simulink model "CLSfixedExample1"  (R2025b)
settings: Solver=FixedStepAuto  StartTime=0.0  StopTime=10  FixedStep=0.0005  RelTol=1e-3
undefined symbols (not defined in the file): AVI, BCL, cfg_length, f1, f2, LRI, pNode_length, pPath_length, PVARP, SD, sig1, sig2, stepsize, URI, VR, VRP, VT
libraries: Libs x8, Libs_unified x3
settings Model: SimulationMode=accelerator  Creator=ball907  LastModifiedBy=rfen801
settings SolverCC: AutoInsertRateTranBlk=on
settings OptimizationCC: DefaultParameterBehavior=Inlined
settings ModelReferenceCC: EnableRefExpFcnMdlSchedulingChecks=on
settings RTWCC: Toolchain=Simulink Real-Time Toolchain  BuildConfiguration=Faster Runs  CodeExecutionProfiling=on

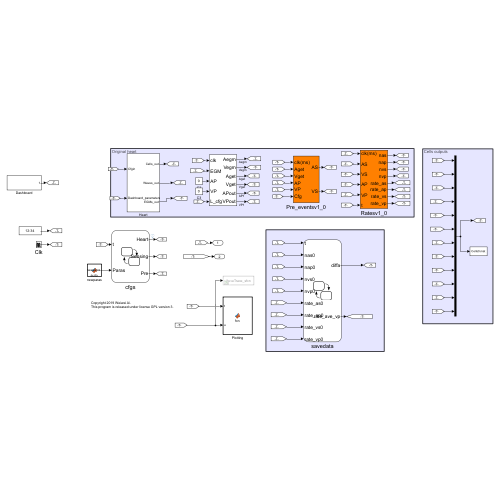
[thumbnail: Simulink's stored preview of the top-level diagram]
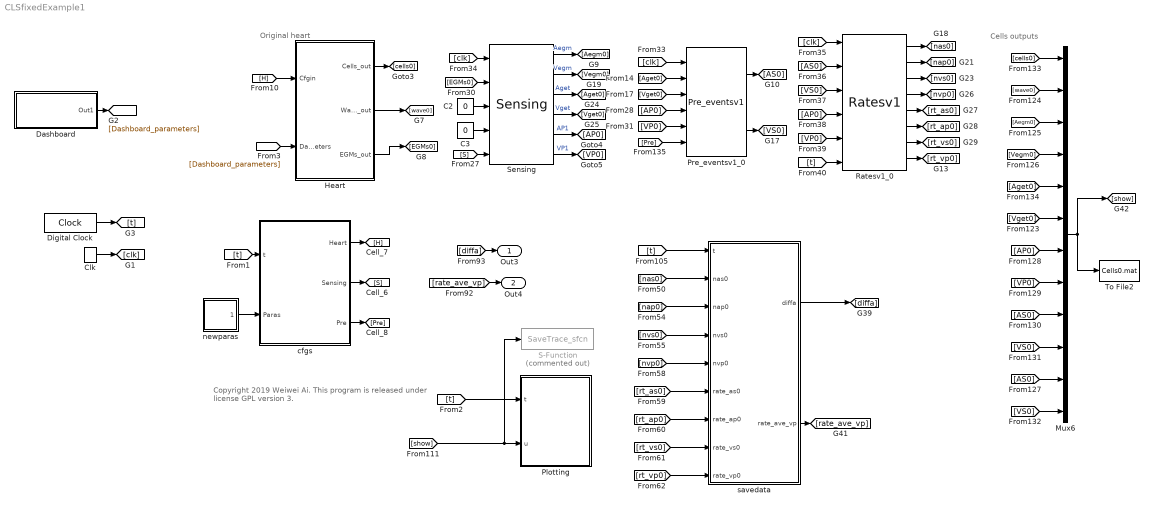
== system CLSfixedExample1 ==
  note: Cells outputs
  note: Copyright 2019 Weiwei Ai.
      | This program is released under license GPL version 3.
  note: Original heart
  C2 : Constant  Value=0
  C3 : Constant  Value=0
  Clk : DiscretePulseGenerator  PulseType=Time based  Period=1  PulseWidth=50
  Dashboard : Subsystem
  Digital Clock : DigitalClock  SampleTime=stepsize
  Heart : Subsystem
  Mux6 : Mux  Inputs=12
  Plotting : MATLAB Function  TreatAsAtomicUnit=on  SystemSampleTime=stepsize*5
  Pre_eventsv1_0 : Libs_unified/Pre_eventsv1  SystemSampleTime=-1  VariantActivationTime=update diagram  EmptyChoice=off  PassThrough=off  PassThroughVariantControl=(default)  EmptyChoiceVariantControl=(default)  AllowFlexibleInterface=on  Latency=0  AutoFrameSizeCalculation=off
  Ratesv1_0 : Libs_unified/Ratesv1  SystemSampleTime=-1  VariantActivationTime=update diagram  EmptyChoice=off  PassThrough=off  PassThroughVariantControl=(default)  EmptyChoiceVariantControl=(default)  AllowFlexibleInterface=on  Latency=0  AutoFrameSizeCalculation=off
  S-Function : S-Function  Commented=on  FunctionName=SaveTrace_sfcn  Parameters=1  SFunctionDeploymentMode=off  EnableBusSupport=off
  Sensing : Libs_unified/Sensing  SystemSampleTime=-1  VariantActivationTime=update diagram  EmptyChoice=off  PassThrough=off  PassThroughVariantControl=(default)  EmptyChoiceVariantControl=(default)  AllowFlexibleInterface=on  Latency=0  AutoFrameSizeCalculation=off
  To File2 : ToFile  Filename=Cells0.mat  MatrixName=cells
      settings: Decimation=2
  cfgs : Stateflow chart  TreatAsAtomicUnit=on
  newparas : MATLAB Function  TreatAsAtomicUnit=on
  savedata : Stateflow chart  TreatAsAtomicUnit=on
  Out3 : Outport
  Out4 : Outport  Port=2
  wires:
  Sensing/6 -> [VP0]  "VP1"
  [VS0] -> Mux6/10
  [VS0] -> Ratesv1_0/3
  Pre_eventsv1_0/1 -> [AS0]
  [nap0] -> savedata/3(nap0)
  [VP0] -> Pre_eventsv1_0/5
  [AS0] -> Mux6/11
  Sensing/3 -> [Aget0]  "Aget"
  [rt_ap0] -> savedata/7(rate_ap0)
  C3/1 -> Sensing/4
  [AS0] -> Mux6/9
  Sensing/1 -> [Aegm0]  "Aegm"
  Ratesv1_0/4 -> [nvp0]
  [t] -> savedata/1(t)
  savedata/1(diffa) -> [diffa]
  Heart/3(EGMs_out) -> [EGMs0]
  [cells0] -> Mux6/1
  Pre_eventsv1_0/2 -> [VS0]
  Sensing/4 -> [Vget0]  "Vget"
  Ratesv1_0/5 -> [rt_as0]
  Ratesv1_0/3 -> [nvs0]
  [rt_vp0] -> savedata/9(rate_vp0)
  [rt_vs0] -> savedata/8(rate_vs0)
  [Aget0] -> Pre_eventsv1_0/2
  Sensing/5 -> [AP0]  "AP1"
  Ratesv1_0/1 -> [nas0]
  [diffa] -> Out3/1
  Heart/1(Cells_out) -> [cells0]
  Ratesv1_0/2 -> [nap0]
  [VP0] -> Mux6/8
  Mux6/1 -> [show], To File2/1
  [AS0] -> Ratesv1_0/2
  [AP0] -> Mux6/7
  [t] -> Ratesv1_0/6
  [Aegm0] -> Mux6/3
  [nvs0] -> savedata/4(nvs0)
  [Vget0] -> Mux6/6
  [rt_as0] -> savedata/6(rate_as0)
  [VS0] -> Mux6/12
  [AP0] -> Ratesv1_0/4
  Heart/2(Waves_out) -> [wave0]
  [clk] -> Ratesv1_0/1
  [clk] -> Pre_eventsv1_0/1
  [Pre] -> Pre_eventsv1_0/6
  [Vget0] -> Pre_eventsv1_0/3
  [wave0] -> Mux6/2
  [VP0] -> Ratesv1_0/5
  [AP0] -> Pre_eventsv1_0/4
  savedata/2(rate_ave_vp) -> [rate_ave_vp]
  C2/1 -> Sensing/3
  [S] -> Sensing/5
  [rate_ave_vp] -> Out4/1
  Ratesv1_0/7 -> [rt_vs0]
  [Vegm0] -> Mux6/4
  [clk] -> Sensing/1
  Ratesv1_0/8 -> [rt_vp0]
  [Aget0] -> Mux6/5
  [nas0] -> savedata/2(nas0)
  [EGMs0] -> Sensing/2
  Sensing/2 -> [Vegm0]  "Vegm"
  Ratesv1_0/6 -> [rt_ap0]
  [nvp0] -> savedata/5(nvp0)
  cfgs/2(Sensing) -> [S]
  cfgs/3(Pre) -> [Pre]
  newparas/1(newparas) -> cfgs/2(Paras)
  cfgs/1(Heart) -> [H]
  [t] -> cfgs/1(t)
  Digital Clock/1 -> [t]
  Clk/1 -> [clk]
  [show] -> S-Function/1, Plotting/2(u)
  [t] -> Plotting/1(t)
  [H] -> Heart/1(Cfgin)
  [Dashboard_parameters] -> Heart/2(Dashboard_parameters)
  Dashboard/1(Out1) -> [Dashboard_parameters]

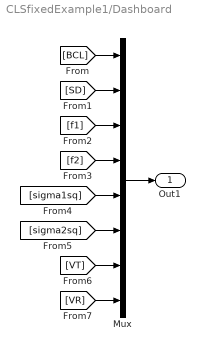
== system CLSfixedExample1/Dashboard ==
  Mux : Mux  Inputs=8
  Out1 : Outport
  wires:
  Mux/1 -> Out1/1
  [BCL] -> Mux/1
  [SD] -> Mux/2
  [f1] -> Mux/3
  [f2] -> Mux/4
  [sigma1sq] -> Mux/5
  [sigma2sq] -> Mux/6
  [VT] -> Mux/7
  [VR] -> Mux/8

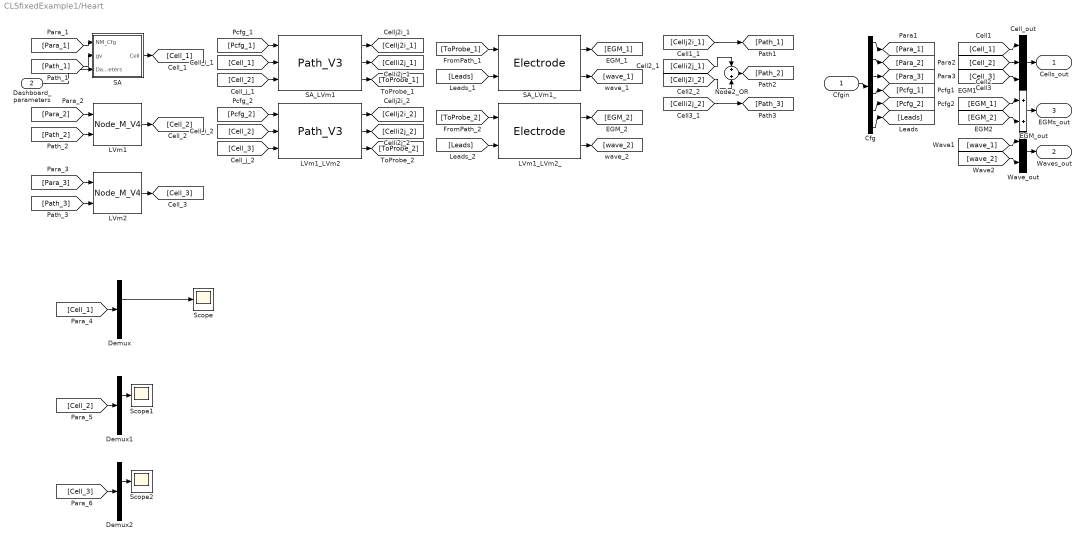
== system CLSfixedExample1/Heart ==
  Cfgin : Inport
  Dashboard_parameters : Inport  Port=2
  Cell_out : Mux  Inputs=3
  Cfg : Demux  Outputs=[50,25,25,11,11,28]
  Demux : Demux  Outputs=5
  Demux1 : Demux  Outputs=5
  Demux2 : Demux  Outputs=5
  EGM_out : Sum  Inputs=2
  LVm1 : Libs/Node_M_V4  SystemSampleTime=-1  VariantActivationTime=update diagram  EmptyChoice=off  PassThrough=off  PassThroughVariantControl=(default)  EmptyChoiceVariantControl=(default)  AllowFlexibleInterface=on  Latency=0  AutoFrameSizeCalculation=off
  LVm1_LVm2 : Libs/Path_V3  SystemSampleTime=-1  VariantActivationTime=update diagram  EmptyChoice=off  PassThrough=off  PassThroughVariantControl=(default)  EmptyChoiceVariantControl=(default)  AllowFlexibleInterface=on  Latency=0  AutoFrameSizeCalculation=off
  LVm1_LVm2_ : Libs/Electrode  SystemSampleTime=-1  VariantActivationTime=update diagram  EmptyChoice=off  PassThrough=off  PassThroughVariantControl=(default)  EmptyChoiceVariantControl=(default)  AllowFlexibleInterface=on  Latency=0  AutoFrameSizeCalculation=off
  LVm2 : Libs/Node_M_V4  SystemSampleTime=-1  VariantActivationTime=update diagram  EmptyChoice=off  PassThrough=off  PassThroughVariantControl=(default)  EmptyChoiceVariantControl=(default)  AllowFlexibleInterface=on  Latency=0  AutoFrameSizeCalculation=off
  Node2_OR : Sum  Inputs=2
  SA : Subsystem  AncestorBlock=Libs/Node_NM_V4
  SA_LVm1 : Libs/Path_V3  SystemSampleTime=-1  VariantActivationTime=update diagram  EmptyChoice=off  PassThrough=off  PassThroughVariantControl=(default)  EmptyChoiceVariantControl=(default)  AllowFlexibleInterface=on  Latency=0  AutoFrameSizeCalculation=off
  SA_LVm1_ : Libs/Electrode  SystemSampleTime=-1  VariantActivationTime=update diagram  EmptyChoice=off  PassThrough=off  PassThroughVariantControl=(default)  EmptyChoiceVariantControl=(default)  AllowFlexibleInterface=on  Latency=0  AutoFrameSizeCalculation=off
  Scope : Scope
      settings: ActiveDisplayYMinimum=-15.358773094825372  ActiveDisplayYMaximum=138.22895785342837
  Scope1 : Scope
      settings: ActiveDisplayYMinimum=-15.358773094825372  ActiveDisplayYMaximum=138.22895785342837
  Scope2 : Scope
      settings: ActiveDisplayYMinimum=-15.358773094825372  ActiveDisplayYMaximum=138.22895785342837  DataLoggingVariableName=ScopeData2
  Wave_out : Mux  Inputs=2
  Cells_out : Outport
  Waves_out : Outport  Port=2
  EGMs_out : Outport  Port=3
  wires:
  [wave_2] -> Wave_out/2
  [wave_1] -> Wave_out/1
  [EGM_2] -> EGM_out/2
  [EGM_1] -> EGM_out/1
  [Cell_3] -> Cell_out/3
  [Cell_2] -> Cell_out/2
  [Cell_1] -> Cell_out/1
  Wave_out/1 -> Waves_out/1
  EGM_out/1 -> EGMs_out/1
  Cell_out/1 -> Cells_out/1
  Cfg/6 -> [Leads]
  Cfg/5 -> [Pcfg_2]
  Cfg/4 -> [Pcfg_1]
  Cfg/3 -> [Para_3]
  Cfg/2 -> [Para_2]
  Cfg/1 -> [Para_1]
  Cfgin/1 -> Cfg/1
  [Celli2j_2] -> [Path_3]
  Node2_OR/1 -> [Path_2]
  [Cellj2i_2] -> Node2_OR/2
  [Celli2j_1] -> Node2_OR/1
  [Cellj2i_1] -> [Path_1]
  [Leads] -> LVm1_LVm2_/2
  [ToProbe_2] -> LVm1_LVm2_/1
  LVm1_LVm2_/2 -> [wave_2]
  LVm1_LVm2_/1 -> [EGM_2]
  [Leads] -> SA_LVm1_/2
  [ToProbe_1] -> SA_LVm1_/1
  SA_LVm1_/2 -> [wave_1]
  SA_LVm1_/1 -> [EGM_1]
  [Cell_3] -> LVm1_LVm2/3
  [Cell_2] -> LVm1_LVm2/2
  [Pcfg_2] -> LVm1_LVm2/1
  LVm1_LVm2/3 -> [ToProbe_2]
  LVm1_LVm2/2 -> [Celli2j_2]
  LVm1_LVm2/1 -> [Cellj2i_2]
  [Cell_2] -> SA_LVm1/3
  [Cell_1] -> SA_LVm1/2
  [Pcfg_1] -> SA_LVm1/1
  SA_LVm1/3 -> [ToProbe_1]
  SA_LVm1/2 -> [Celli2j_1]
  SA_LVm1/1 -> [Cellj2i_1]
  [Path_3] -> LVm2/2
  [Para_3] -> LVm2/1
  LVm2/1 -> [Cell_3]
  [Path_2] -> LVm1/2
  [Para_2] -> LVm1/1
  LVm1/1 -> [Cell_2]
  [Path_1] -> SA/2(gv)
  [Para_1] -> SA/1(NM_Cfg)
  SA/1(Cell) -> [Cell_1]
  [Cell_1] -> Demux/1
  Demux/2 -> Scope/1
  [Cell_2] -> Demux1/1
  Demux1/2 -> Scope1/1
  [Cell_3] -> Demux2/1
  Demux2/2 -> Scope2/1
  Dashboard_parameters/1 -> SA/3(Dashboard_parameters)

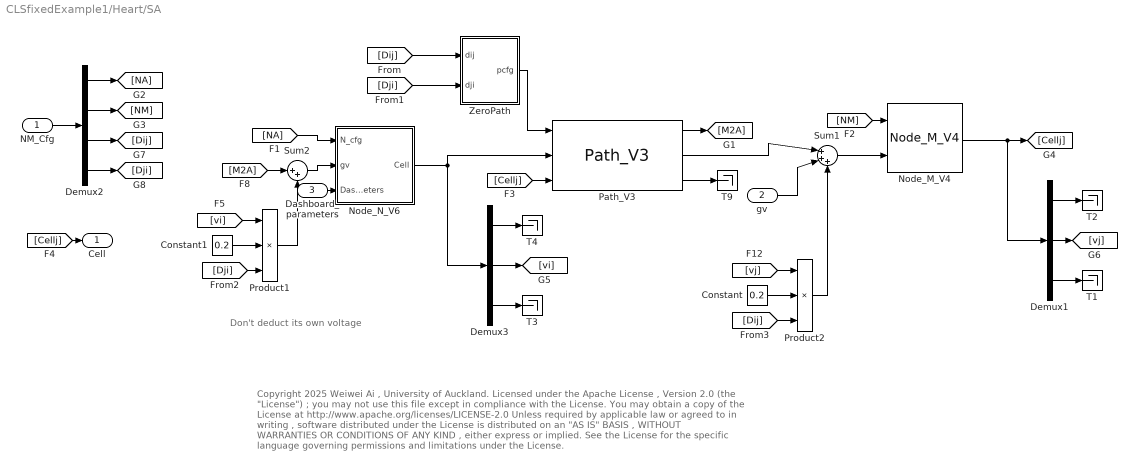
== system CLSfixedExample1/Heart/SA ==
  note: Copyright 2025 Weiwei Ai , University of Auckland.
      | Licensed under the Apache License , Version 2.0 (the "License") ;
      | you may not use this file except in compliance with the License.
      | You may obtain a copy of the License at
      | http://www.apache.org/licenses/LICENSE-2.0
      | Unless required by applicable law or agreed to in writing , software
      | distributed under the License is distributed on an "AS IS" BASIS ,
      | WITHOUT WARRANTIES OR CONDITIONS OF ANY KIND , either express or implied.
      | See the License for the specific language governing permissions and
      | limitations under the License.
  note: Don't deduct its own voltage
  NM_Cfg : Inport
  gv : Inport  Port=2
  Dashboard_parameters : Inport  Port=3
  Constant : Constant  Value=0.2
  Constant1 : Constant  Value=0.2
  Demux1 : Demux  Outputs=[1,1,3]
  Demux2 : Demux  Outputs=[23,25,1,1]
  Demux3 : Demux  Outputs=[1,1,3]
  Node_M_V4 : Libs/Node_M_V4  SystemSampleTime=-1  VariantActivationTime=update diagram  EmptyChoice=off  PassThrough=off  PassThroughVariantControl=(default)  EmptyChoiceVariantControl=(default)  AllowFlexibleInterface=on  Latency=0  AutoFrameSizeCalculation=off
  Node_N_V6 : Subsystem  AncestorBlock=Libs/Node_N_V6
  Path_V3 : Libs/Path_V3  SystemSampleTime=-1  VariantActivationTime=update diagram  EmptyChoice=off  PassThrough=off  PassThroughVariantControl=(default)  EmptyChoiceVariantControl=(default)  AllowFlexibleInterface=on  Latency=0  AutoFrameSizeCalculation=off
  Product1 : Product  Inputs=***
  Product2 : Product  Inputs=***
  Sum1 : Sum  Inputs=|+++
  Sum2 : Sum  Inputs=|++
  T{1..4,9} (5 alike) : Terminator
  ZeroPath : MATLAB Function  TreatAsAtomicUnit=on
  Cell : Outport
  wires:
  [Dij] -> Product2/3
  [Dji] -> Product1/3
  [Dji] -> ZeroPath/2(dji)
  [Dij] -> ZeroPath/1(dij)
  Demux2/4 -> [Dji]
  Demux2/3 -> [Dij]
  Product1/1 -> Sum2/2
  [vi] -> Product1/1
  Constant1/1 -> Product1/2
  Sum2/1 -> Node_N_V6/2(gv)
  [M2A] -> Sum2/1
  gv/1 -> Sum1/2
  Product2/1 -> Sum1/3
  [vj] -> Product2/1
  Constant/1 -> Product2/2
  Demux1/2 -> [vj]
  Demux3/2 -> [vi]
  Demux3/1 -> T4/1
  Demux3/3 -> T3/1
  Node_N_V6/1(Cell) -> Demux3/1, Path_V3/2
  Demux1/1 -> T2/1
  Demux1/3 -> T1/1
  Sum1/1 -> Node_M_V4/2
  Path_V3/2 -> Sum1/1
  ZeroPath/1(pcfg) -> Path_V3/1
  [Cellj] -> Cell/1
  [Cellj] -> Path_V3/3
  Node_M_V4/1 -> [Cellj], Demux1/1
  Path_V3/1 -> [M2A]
  [NM] -> Node_M_V4/1
  [NA] -> Node_N_V6/1(N_cfg)
  Demux2/2 -> [NM]
  Demux2/1 -> [NA]
  Path_V3/3 -> T9/1
  NM_Cfg/1 -> Demux2/1
  Dashboard_parameters/1 -> Node_N_V6/3(Dashboard_parameters)

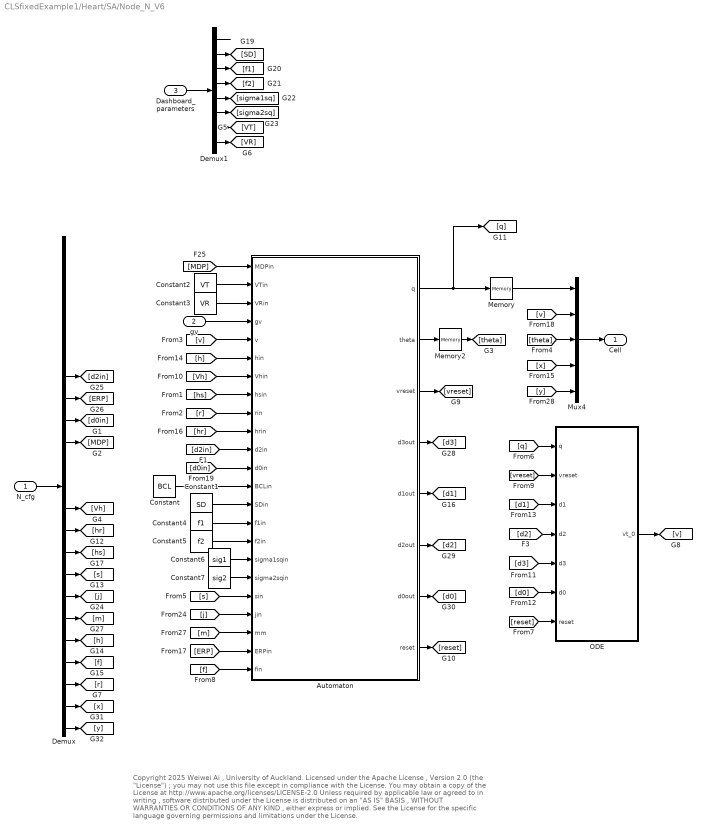
== system CLSfixedExample1/Heart/SA/Node_N_V6 ==
  note: Copyright 2025 Weiwei Ai , University of Auckland.
      | Licensed under the Apache License , Version 2.0 (the "License") ;
      | you may not use this file except in compliance with the License.
      | You may obtain a copy of the License at
      | http://www.apache.org/licenses/LICENSE-2.0
      | Unless required by applicable law or agreed to in writing , software
      | distributed under the License is distributed on an "AS IS" BASIS ,
      | WITHOUT WARRANTIES OR CONDITIONS OF ANY KIND , either express or implied.
      | See the License for the specific language governing permissions and
      | limitations under the License.
  N_cfg : Inport
  gv : Inport  Port=2
  Dashboard_parameters : Inport  Port=3
  Automaton : Stateflow chart  TreatAsAtomicUnit=on
  Constant : Constant  Value=BCL
  Constant1 : Constant  Value=SD
  Constant2 : Constant  Value=VT
  Constant3 : Constant  Value=VR
  Constant4 : Constant  Value=f1
  Constant5 : Constant  Value=f2
  Constant6 : Constant  Value=sig1
  Constant7 : Constant  Value=sig2
  Demux : Demux  Outputs=23
  Demux1 : Demux  Outputs=8
  Memory : Memory
  Memory2 : Memory
  Mux4 : Mux  Inputs=5
  ODE : Subsystem
  Cell : Outport
  wires:
  gv/1 -> Automaton/4(gv)
  [y] -> Mux4/5
  [x] -> Mux4/4
  Demux/23 -> [y]
  Demux/22 -> [x]
  Automaton/7(d0out) -> [d0]
  Automaton/6(d2out) -> [d2]
  [f] -> Automaton/23(fin)
  Automaton/4(d3out) -> [d3]
  [ERP] -> Automaton/22(ERPin)
  [m] -> Automaton/21(mm)
  Demux/18 -> [m]
  Demux/19 -> [h]
  Demux/20 -> [f]
  Demux/21 -> [r]
  Demux/17 -> [j]
  [j] -> Automaton/20(jin)
  [s] -> Automaton/19(sin)
  Demux/13 -> [Vh]
  Demux/14 -> [hr]
  Demux/15 -> [hs]
  Demux/16 -> [s]
  Demux/10 -> [MDP]
  Demux/9 -> [d0in]
  Demux/8 -> [ERP]
  Demux/7 -> [d2in]
  Constant7/1 -> Automaton/18(sigma2sqin)
  Constant6/1 -> Automaton/17(sigma1sqin)
  Constant5/1 -> Automaton/16(f2in)
  Constant4/1 -> Automaton/15(f1in)
  Constant1/1 -> Automaton/14(SDin)
  Constant/1 -> Automaton/13(BCLin)
  [d0in] -> Automaton/12(d0in)
  [d2in] -> Automaton/11(d2in)
  Automaton/5(d1out) -> [d1]
  Memory2/1 -> [theta]
  Automaton/2(theta) -> Memory2/1
  [theta] -> Mux4/3
  [v] -> Mux4/2
  [hr] -> Automaton/10(hrin)
  [h] -> Automaton/6(hin)
  [hs] -> Automaton/8(hsin)
  [Vh] -> Automaton/7(Vhin)
  [vreset] -> ODE/2(vreset)
  [reset] -> ODE/7(reset)
  [q] -> ODE/1(q)
  Automaton/8(reset) -> [reset]
  Automaton/3(vreset) -> [vreset]
  ODE/1(vt_0) -> [v]
  [v] -> Automaton/5(v)
  [d0] -> ODE/6(d0)
  [d3] -> ODE/5(d3)
  [d2] -> ODE/4(d2)
  [d1] -> ODE/3(d1)
  [r] -> Automaton/9(rin)
  [MDP] -> Automaton/1(MDPin)
  Constant2/1 -> Automaton/2(VTin)
  Constant3/1 -> Automaton/3(VRin)
  Memory/1 -> Mux4/1
  Mux4/1 -> Cell/1
  Automaton/1(q) -> [q], Memory/1
  N_cfg/1 -> Demux/1
  Demux1/1 -> ?
  Demux1/2 -> [SD]
  Demux1/3 -> [f1]
  Demux1/4 -> [f2]
  Demux1/5 -> [sigma1sq]
  Demux1/6 -> [sigma2sq]
  Demux1/7 -> [VT]
  Demux1/8 -> [VR]
  Dashboard_parameters/1 -> Demux1/1

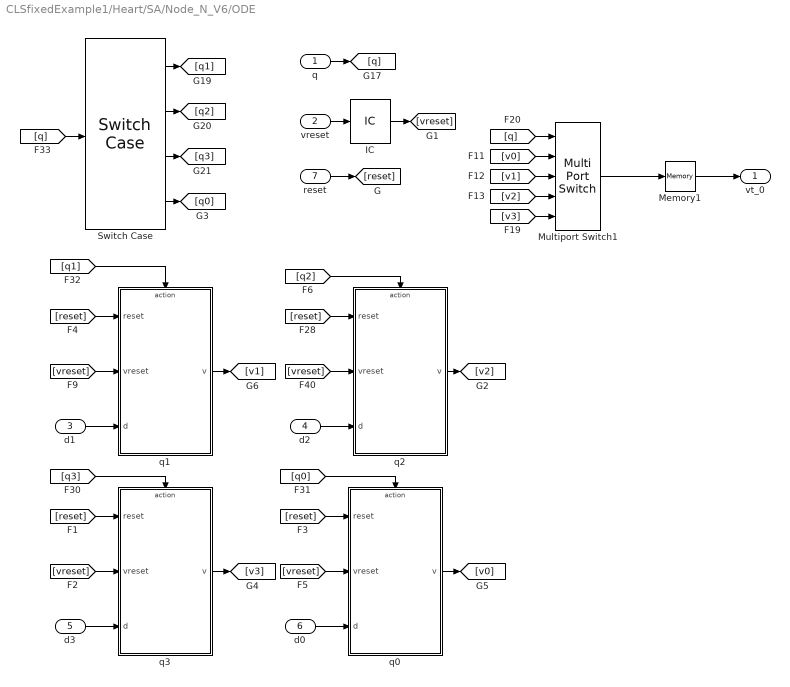
== system CLSfixedExample1/Heart/SA/Node_N_V6/ODE ==
  q : Inport
  vreset : Inport  Port=2
  d1 : Inport  Port=3
  d2 : Inport  Port=4
  d3 : Inport  Port=5
  d0 : Inport  Port=6
  reset : Inport  Port=7
  IC : InitialCondition  Value=0
  Memory1 : Memory
  Multiport Switch1 : MultiPortSwitch  DataPortOrder=Zero-based contiguous  Inputs=4  zeroidx=on  SaturateOnIntegerOverflow=off  InputSameDT=off
  Switch Case : SwitchCase  CaseConditions={1,2,3,0}  ShowDefaultCase=off
  q0 : Subsystem  TreatAsAtomicUnit=on
  q1 : Subsystem  TreatAsAtomicUnit=on
  q2 : Subsystem  TreatAsAtomicUnit=on
  q3 : Subsystem  TreatAsAtomicUnit=on
  vt_0 : Outport
  wires:
  d1/1 -> q1/3(d)
  [vreset] -> q1/2(vreset)
  [reset] -> q2/1(reset)
  [v3] -> Multiport Switch1/5
  [v2] -> Multiport Switch1/4
  [v1] -> Multiport Switch1/3
  [v0] -> Multiport Switch1/2
  Memory1/1 -> vt_0/1
  [q0] -> q0/Action
  [q3] -> q3/Action
  [vreset] -> q0/2(vreset)
  [reset] -> q0/1(reset)
  d0/1 -> q0/3(d)
  q0/1(v) -> [v0]
  [vreset] -> q3/2(vreset)
  [reset] -> q3/1(reset)
  d3/1 -> q3/3(d)
  q3/1(v) -> [v3]
  [vreset] -> q2/2(vreset)
  [q2] -> q2/Action
  d2/1 -> q2/3(d)
  q2/1(v) -> [v2]
  Switch Case/4 -> [q0]
  Switch Case/3 -> [q3]
  Switch Case/2 -> [q2]
  Switch Case/1 -> [q1]
  [reset] -> q1/1(reset)
  [q1] -> q1/Action
  [q] -> Switch Case/1
  [q] -> Multiport Switch1/1
  q1/1(v) -> [v1]
  q/1 -> [q]
  reset/1 -> [reset]
  vreset/1 -> IC/1
  IC/1 -> [vreset]
  Multiport Switch1/1 -> Memory1/1

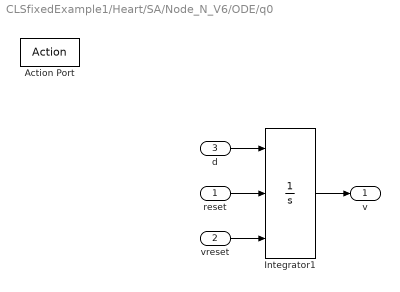
== system CLSfixedExample1/Heart/SA/Node_N_V6/ODE/q0 ==
  reset : Inport
  vreset : Inport  Port=2
  d : Inport  Port=3
  Action Port : ActionPort  InitializeStates=reset  ActionPortLabel=case [ 0 ]:
  Integrator1 : Integrator  ExternalReset=either  InitialConditionSource=external  InitialCondition=20
  v : Outport
  wires:
  Integrator1/1 -> v/1
  reset/1 -> Integrator1/2
  vreset/1 -> Integrator1/3
  d/1 -> Integrator1/1

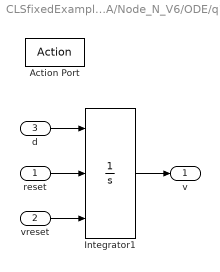
== system CLSfixedExample1/Heart/SA/Node_N_V6/ODE/q1 ==
  reset : Inport
  vreset : Inport  Port=2
  d : Inport  Port=3
  Action Port : ActionPort  InitializeStates=reset  ActionPortLabel=case [ 1 ]:
  Integrator1 : Integrator  ExternalReset=either  InitialConditionSource=external  InitialCondition=20
  v : Outport
  wires:
  d/1 -> Integrator1/1
  Integrator1/1 -> v/1
  reset/1 -> Integrator1/2
  vreset/1 -> Integrator1/3

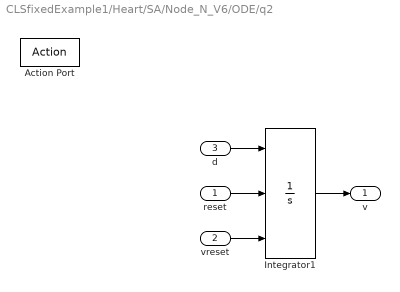
== system CLSfixedExample1/Heart/SA/Node_N_V6/ODE/q2 ==
  reset : Inport
  vreset : Inport  Port=2
  d : Inport  Port=3
  Action Port : ActionPort  InitializeStates=reset  ActionPortLabel=case [ 2 ]:
  Integrator1 : Integrator  ExternalReset=either  InitialConditionSource=external  InitialCondition=20
  v : Outport
  wires:
  d/1 -> Integrator1/1
  vreset/1 -> Integrator1/3
  reset/1 -> Integrator1/2
  Integrator1/1 -> v/1

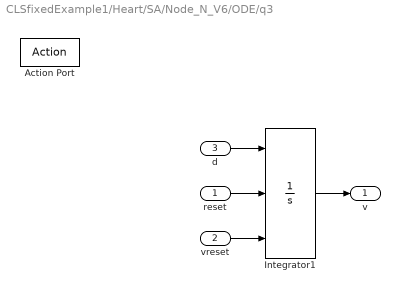
== system CLSfixedExample1/Heart/SA/Node_N_V6/ODE/q3 ==
  reset : Inport
  vreset : Inport  Port=2
  d : Inport  Port=3
  Action Port : ActionPort  InitializeStates=reset  ActionPortLabel=case [ 3 ]:
  Integrator1 : Integrator  ExternalReset=either  InitialConditionSource=external  InitialCondition=20
  v : Outport
  wires:
  Integrator1/1 -> v/1
  reset/1 -> Integrator1/2
  vreset/1 -> Integrator1/3
  d/1 -> Integrator1/1

== stateflow chart CLSfixedExample1/cfgs ==
  settings: executeAtInitialization=1
  state Ini
  state wait
  Ini -> wait : [t>800]{pUpdate(Paras);}
  (default) -> Ini : {Sensing=Scfgf;[Pre]=Precfg;...
      |  [Heart] =LoadInit;}
  data: Scfg function_output; Preout function_output; LRI parameter; AVI parameter; VRP parameter; URI parameter; PVARP parameter; Parasin function_input; pNode_length parameter; pPath_length parameter; Hcfg function_output; cfg_length parameter; Heart output; Sensing output; t input; Paras input; Pre output
  function Scfg= Scfgf:
    | function Scfg= Scfgf
    | 
    | %% desired
    | xa=1;
    | xc=0.05;
    | xc1=0.1;
    | xd=1;
    | xe=0.1;
    | avd=100;
    | vad=100;
    | uni_a=1;
    | Sens_a=0.6;
    | Amp_ap=500;
    | uni_v=1;
    | Sens_v=2.8;
    | Amp_vp=500;
    | 
    | Scfg=[xa xc xc1 xd xe avd vad uni_a Sens_a Amp_ap uni_v Sens_v Amp_vp]';
    | 
    | end
  function Preout = Precfg:
    | function Preout = Precfg
    | % 
    | % LRI=1000;
    | % AVI=170;
    | % URI=500;
    | % VRP=230;
    | % PVARP=250;
    | Preout=[VRP PVARP];
    | 
    | end
  function pUpdate(Parasin):
    | %% Get the index of the parameter
    | function pUpdate(Parasin)
    | %#codegen
    | coder.extrinsic('evalin');
    | coder.extrinsic('assignin');
    | Nodein=zeros(1,pNode_length); % The total number of cell cfg ports
    | Nodein=evalin('base', 'pNode');
    | Pathin=zeros(1,pPath_length); % The total number of path cfg ports
    | Pathin=evalin('base', 'pPath');
    | for n=1:pNode_length
    |     m=Nodein(n);
    |     Heart(m)=Parasin(n);
    | end
    | 
    | for n=1:pPath_length
    |     m=Pathin(n);
    |     nn=n+length(Nodein);
    |     Heart(m)=Parasin(nn);
    | end
    | 
    | assignin('base', 'Params', Parasin);
    | 
    | end
  function Hcfg   = LoadInit:
    | function Hcfg   = LoadInit
    | %#codegen
    | coder.extrinsic('evalin');
    | Hcfg1=zeros(1,cfg_length); % The total number of cfg ports
    | Hcfg1=evalin('base', 'cfgdata');
    | Hcfg=Hcfg1';
    | end

== matlab function CLSfixedExample1/Plotting ==
  data: t input; u input
function fcn(t,u)
%coder.extrinsic('evalin')
coder.extrinsic('updateGUIplots')
fun = 'updateGUIplots';
updateGUIplots(t,u)
%feval(fun,t,u)
end

== matlab function CLSfixedExample1/Heart/SA/ZeroPath ==
  data: pcfg output; dij input; dji input
function pcfg= Path(dij,dji)
%#codegen
CVi2j=1;
Dij=dij;
aij=1;
bij=0;
cij=0;

CVj2i=1;
Dji=dji;
aji=1;
bji=0;
cji=0;
C=5;

pcfg=[CVi2j,Dij, aij, bij, cij,CVj2i,Dji, aji,bji,cji,C];
end

== matlab function CLSfixedExample1/newparas ==
  data: newparas output; paras_length parameter

function newparas= auto(paras_length)

coder.extrinsic('evalin');
%par_length = evalin('base','paras_length')
newparas=zeros(1,paras_length); % The total number of cell cfg ports
newparas=evalin('base', 'pp');

end

== stateflow chart CLSfixedExample1/savedata ==
  settings: executeAtInitialization=1
  state termi
  state difa
  state Ini
  difa -> termi [order 1] : [rate_ave_a0>=60]/{coder.extrinsic('assignin');diffa=rate_ave_a1-rate_ave_a0;assignin('base', 'diffa', diffa);}
  (default) -> Ini : {rate_ave_vp=0; diffa=0;}
  Ini -> difa : [t>=29998]{coder.extrinsic('assignin','mean');...
      | assignin('base', 'nas0', nas0);assignin('base', 'nap0', nap0);assignin('base', 'nvs0', nvs0);assignin('base', 'nvp0', nvp0);...
      | assignin('base', 'rate_as0', rate_as0);assignin('base', 'rate_ap0', rate_ap0);assignin('base', 'rate_vs0', rate_vs0);assignin('base', 'rate_vp0', rate_vp0);...
      | rate_ave_vp=mean(rate_vp0(2,1:nvp0));assignin('base', 'rate_ave_vp', rate_ave_vp);...
      | rate_ave_a1=0;rate_ave_a0=0;rate_ave_a0=mean(rate_as0(2,1:nas0));rate_ave_a1=zeros(size(rate_ave_a0),like=rate_ave_a0);}
  difa -> termi [order 2] : [rate_ave_a0<60]/{coder.extrinsic('assignin');diffa=rate_ave_a1-60;assignin('base', 'diffa', diffa);}
  data: t input; nas0 input; nap0 input; nvs0 input; nvp0 input; rate_as0 input; rate_ap0 input; rate_vs0 input; rate_vp0 input; diffa output double; rate_ave_vp output double; rate_ave_a0 local double; rate_ave_a1 local double

== stateflow chart CLSfixedExample1/Heart/SA/Node_N_V6/Automaton ==
  settings: updateMethod=DISCRETE
  state PacemakerCell
    state Cell [parallel]
      settings: executionOrder=1
      state Slow
        en: q=1; %phase4
      state Stimulated
        en: q=2; %phase0
        f1theta=exp(-h*theta);
        Vmax=(-1)*MDP*f1theta;
        [f3theta,n,Vmin]=sat(n,hr,hs,Vh1,s,m,theta);
      state Plateau
        en: q=3;%phase2
      state RP
        en:q=0;%phase3
      (default) -> Slow : /{Vmin=0;Vmax=(-1)*MDP; d3=d3fcn(MDP,VR,VT,d0,d2,ERP); BCL=RR(BCLin,SDin,f1in,f2in,sigma1sqin,sigma2sqin,t);...
          | t3=(abs(MDP)-VR)/abs(d3); t0=VR/abs(d0);t2=(abs(MDP)-VT)/abs(d2);d1=(VT)/(BCL-t3-t0-t2);d1out=d1;}
      Slow -> Stimulated [order 1] : [gv>VT&& v<VT]{theta=(v-VT)/(Vmin-VT);f2theta=exp(-f*theta);d2out=d2*f2theta;...
          |  f4theta=exp(j*(theta-1)); Vh1=Vh*f4theta; n=n+1;  ...
          |  vreset=v;reset; }
      Slow -> Stimulated [order 2] : [v>=VT]{theta=0; f2theta=exp(-f*theta); d2out=d2*f2theta;...
          |  n=(1-r)*n;  vreset=v;reset; }
      RP -> Slow : [v<=Vmin]{t3=(abs(MDP)-VR)/abs(d3); t0=VR/abs(d0);...
          | MDP=MDPin; VT=VTin; d2=d2in; t2=(abs(MDP)-VT)/abs(d2);...
          | BCL=RR(BCLin,SDin,f1in,f2in,sigma1sqin,sigma2sqin,t);...
          | d1=(VT)/(BCL-t3-t0-t2); d1out=d1*f3theta;...
          | VR=VRin; h=hin; Vh=Vhin; hs=hsin; r=rin;hr=hrin;d0=d0in;...
          | s=sin; j=jin; m=mm; ERP=ERPin;f=fin;...
          | vreset=v;reset;}
      Stimulated -> Plateau : [v>=Vmax]{d3=d3fcn(MDP,VR,VT,d0,d2,ERP);...
          | d3out=d3*f2theta;...
          | vreset=v;reset;}
      Plateau -> RP : [v<=VR]{d0out=d0*f2theta; vreset=v;reset;}
    state R [parallel]
      du:
      t=temporalCount(sec);
      settings: executionOrder=2
  (default) -> PacemakerCell : {t=0; MDP=MDPin;VT=VTin;VR=VRin;h=hin;Vh=Vhin;hs=hsin;r=rin;hr=hrin;d2=d2in;d0=d0in;...
      | s=sin;j=jin;m=mm;ERP=ERPin;f=fin;}
  data: f3out function_output double; tout function_output double; pt function_input double; Vminout function_output double; phr function_input double; phs function_input double; pVh function_input double; ps function_input double; pm function_input double; ptheta function_input double; pbcl function_input double; psd function_input double; pf1 function_input double; pf2 function_input double; psigma1sq function_input double; psigma2sq function_input double; rr function_output double size=1; pt function_input double; pMDP function_input double; pVR function_input double; pVT function_input double; pd0 function_input double; pd2 function_input double; pERP function_input double; d3in function_output double; q output double; MDPin input double =0; VTin input double; VRin input; Vmax local double; theta output double; vreset output double; gv input; v input double; hin input double; f1theta local double; Vhin input double; Vh1 local double; hsin input double; rin input double; hrin input double; Vmin local double; d2in input double; d3out output double; d0in input double; BCLin input double; SDin input double; f1in input double; f2in input double; sigma1sqin input double; sigma2sqin input double; d1out output double; Vtemp local double; t local double; sin input double; jin input double; mm input double; ERPin input double; f3theta local double; d2out output double; fin input double; d0out output double; f2theta local double; n local double; f4theta local double; d2 local double; Vh local double; h local double; hr local double; hs local double; j local double; m local double; r local double; s local double; BCL local double; ERP local double; MDP local double; VR local double; VT local double; d0 local double; f local double; d1 local double; d3 local double; t0 local double; t2 local double; t3 local double
  data v settings: updateMethod=SF_CONTINUOUS_TIME_DATA
  events: reset output EITHER_EDGE_EVENT
  function [f3out,tout,Vminout]=sat(pt,phr,phs,pVh,ps,pm,ptheta):
    | function [f3out,tout,Vminout]=sat(pt,phr,phs,pVh,ps,pm,ptheta)
    | 
    | td=phr*(pt-phs);
    | 
    | if td>=5
    |     tout=5/phr+phs;
    | else
    |     tout=pt;
    | end
    | 
    | if tout<1
    | co=0;
    | else
    | Vtemp=1+exp(-phr*(tout-phs)); 
    | co=1/Vtemp;
    | end;
    | Vminout=pVh*co;
    | thetai=ptheta;
    | for i=1:ps-1
    |     thetai=thetai*ptheta;
    | end
    | ft=pm*co*thetai+1;
    | f3out=1/ft;
    | end
  function rr= RR(pbcl,psd,pf1,pf2,psigma1sq,psigma2sq,pt):
    | function rr= RR(pbcl,psd,pf1,pf2,psigma1sq,psigma2sq,pt)
    | %Rate dependent factor
    | c1=0.01;
    | c2=0.01;
    | if psigma1sq<0 || psigma2sq<0
    |     error('Invalid input');
    | end
    | % The Gaussian frequency distribution, power spectrum
    | hf=0.5;
    | fstep=0.025;
    | ff=0:fstep:hf; % The frequency range original;
    | % fmax=1; % Assume the highest frequency
    | % fmin=0.025; % Assume the lowest frequency
    | % Fs=2*fmax; % The sample frequency 
    | % tstep=1/Fs; % The sample period of the time series
    | % tmax=1/fmin; % The period of the time series
    | % N=tmax/tstep;
    | % fstep=2*fmax/N; % =fmin
    | % f=fstep:fstep:fmax; % The frequency range original; 
    | ln=length(ff); % The number of frequency/cos signals.
    | s1=(psigma1sq/(c1*sqrt(2*pi)))*exp(-(ff-pf1).^2/(2*c1^2));
    | s2=(psigma2sq/(c2*sqrt(2*pi)))*exp(-(ff-pf2).^2/(2*c2^2));
    | ss=s1+s2; % s(f)
    | rss=sqrt(ss); %
    | %Construct the time series y(t) from s(f);
    | mag=rss; % the amplitudes;
    | y = ff'*2*pi*pt/1000;
    | y = cos(y);
    | for i=1:ln
    |     y(i,:)=y(i,:)*mag(i);
    | end
    | if ln>1
    |     y1=sum(y);
    | else
    |     y1=y;
    | end
    | rr=pbcl+y1*psd;
    | end
  function d3in= d3fcn(pMDP,pVR,pVT,pd0,pd2,pERP):
    | function d3in= d3fcn(pMDP,pVR,pVT,pd0,pd2,pERP)
    | %#codegen
    | d3in=-(abs(pMDP)-pVR)/(pERP-(abs(pMDP)-pVT)/pd2-pVR/abs(pd0));
